simulink library "Driver_Gamepad_Xbox"  (R2025a)
settings: Solver=VariableStepAuto  StartTime=0.0  StopTime=10.0  RelTol=1e-3
undefined symbols (not defined in the file): Driver
libraries: Gamepad_Xbox x1
Description:
  | Component of Simscape Vehicle Templates Library
  | 
  | Copyright 2018-2025 The MathWorks, Inc.
settings Model: Creator=smiller  LastModifiedBy=smiller
settings SolverCC: AlgebraicLoopSolver=TrustRegion
settings DataIOCC: ReturnWorkspaceOutputs=off
settings DebuggingCC: UnconnectedInputMsg=warning  UnconnectedOutputMsg=warning  UnconnectedLineMsg=warning  ArithmeticOperatorsInVariantConditions=warning
settings ModelReferenceCC: EnableRefExpFcnMdlSchedulingChecks=on
settings SFSimCC: CustomCodeUndefinedFunction=UseInterfaceOnly
settings RTWCC: GPUComputeCapability=3.5  DLArmComputeVersion=19.05

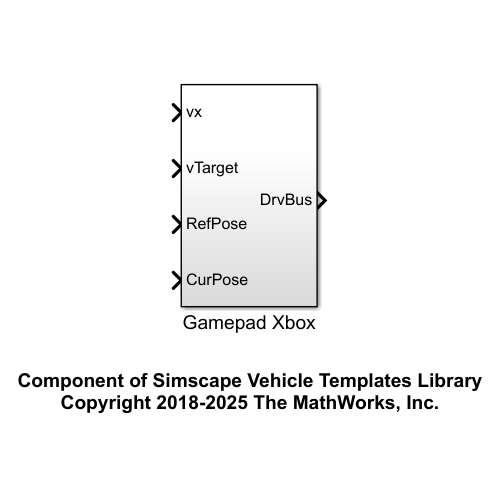
[thumbnail: Simulink's stored preview of the top-level diagram]
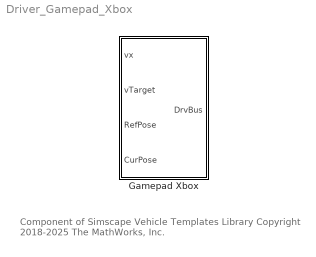
== system Driver_Gamepad_Xbox ==
  note: Component of Simscape Vehicle Templates Library
      | Copyright 2018-2025 The MathWorks, Inc.
  Gamepad Xbox : Subsystem

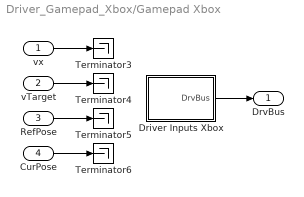
== system Driver_Gamepad_Xbox/Gamepad Xbox ==
  vx : Inport
  vTarget : Inport  Port=2
  RefPose : Inport  Port=3
  CurPose : Inport  Port=4
  Driver Inputs Xbox : Subsystem
  Terminator{3..6} (4 alike) : Terminator
  DrvBus : Outport  VectorParamsAs1DForOutWhenUnconnected=off
  wires:
  Driver Inputs Xbox/1(DrvBus) -> DrvBus/1
  vTarget/1 -> Terminator4/1
  CurPose/1 -> Terminator6/1
  vx/1 -> Terminator3/1
  RefPose/1 -> Terminator5/1

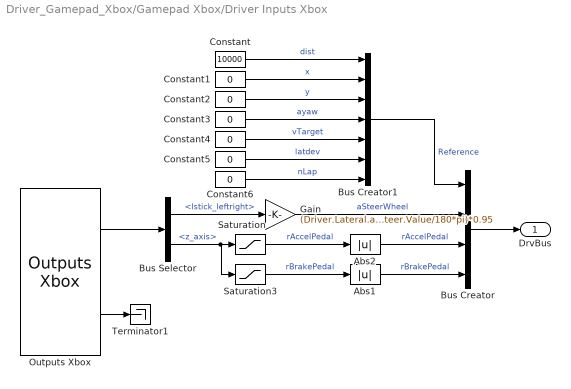
== system Driver_Gamepad_Xbox/Gamepad Xbox/Driver Inputs Xbox ==
  Abs1 : Abs  ZeroCross=off  SaturateOnIntegerOverflow=off
  Abs2 : Abs  ZeroCross=off  SaturateOnIntegerOverflow=off
  Bus Creator : BusCreator  Inputs=4
  Bus Creator1 : BusCreator  Inputs=7
  Bus Selector : BusSelector  OutputSignals=lstick_leftright,z_axis
  Constant : Constant  Value=10000
  Constant{1..6} (6 alike) : Constant  Value=0
  Gain : Gain  Gain=(Driver.Lateral.aMaxSteer.Value/180*pi)*0.95
  Outputs Xbox : Gamepad_Xbox/Outputs Xbox  DLx=0.07  DLy=0.05  Dz=0.01  DRx=0.04  DRy=0.01  joyid=1
  Saturation : Saturate  UpperLimit=0  LowerLimit=-1  ZeroCross=off
  Saturation3 : Saturate  UpperLimit=1  LowerLimit=0  ZeroCross=off
  Terminator1 : Terminator
  DrvBus : Outport  VectorParamsAs1DForOutWhenUnconnected=off
  wires:
  Bus Creator/1 -> DrvBus/1
  Bus Selector/1 -> Gain/1  "<lstick_leftright>"
  Gain/1 -> Bus Creator/2  "aSteerWheel"
  Abs2/1 -> Bus Creator/3  "rAccelPedal"
  Outputs Xbox/1 -> Bus Selector/1
  Abs1/1 -> Bus Creator/4  "rBrakePedal"
  Outputs Xbox/2 -> Terminator1/1
  Saturation3/1 -> Abs1/1  "rBrakePedal"
  Bus Selector/2 -> Saturation/1, Saturation3/1  "<z_axis>"
  Saturation/1 -> Abs2/1  "rAccelPedal"
  Constant3/1 -> Bus Creator1/4  "ayaw"
  Constant/1 -> Bus Creator1/1  "dist"
  Constant4/1 -> Bus Creator1/5  "vTarget"
  Constant1/1 -> Bus Creator1/2  "x"
  Bus Creator1/1 -> Bus Creator/1  "Reference"
  Constant5/1 -> Bus Creator1/6  "latdev"
  Constant2/1 -> Bus Creator1/3  "y"
  Constant6/1 -> Bus Creator1/7  "nLap"
